simulink subsystem "forward_wheel"  (R2024b)
settings: Solver=VariableStepAuto  StartTime=0.0  StopTime=10.0  RelTol=1e-3
undefined symbols (not defined in the file): C_i, J, min_velocity, R
settings Model: Creator=Yevgeniy Gorbachev  LastModifiedBy=Yevgeniy Gorbachev

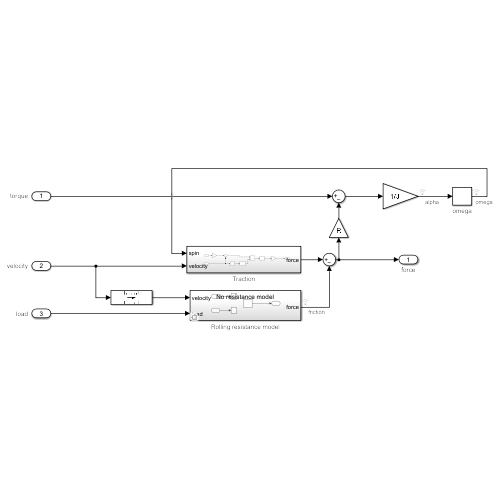
[thumbnail: Simulink's stored preview of the top-level diagram]
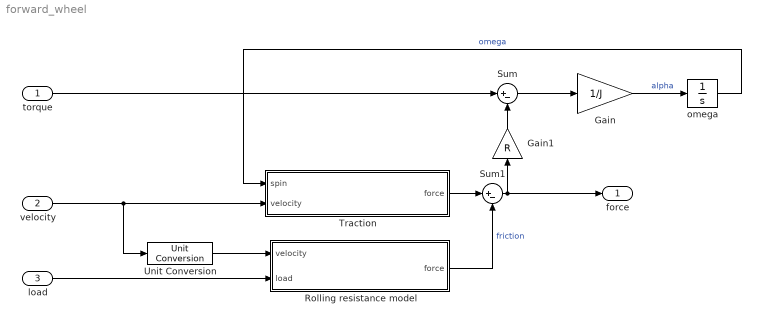
== system forward_wheel ==
  torque : Inport  Unit=N*m@torque  PortDimensions=1
  velocity : Inport  Port=2  Unit=m/s  PortDimensions=1
  load : Inport  Port=3  Unit=N  PortDimensions=1
  Gain : Gain  Gain=1/J
  Gain1 : Gain  Gain=R
  Rolling resistance model : Subsystem  Variant=on  VariantControl=Rolling resistance model
  Sum : Sum  Inputs=|+-
  Sum1 : Sum  Inputs=|+-
  Traction : Subsystem
  Unit Conversion : UnitConversion
  omega : Integrator  InitialCondition=10/R*0
  force : Outport  Unit=N  PortDimensions=1
  wires:
  Sum/1 -> Gain/1
  Gain/1 -> omega/1  "alpha"
  torque/1 -> Sum/1
  velocity/1 -> Unit Conversion/1, Traction/2(velocity)
  omega/1 -> Traction/1(spin)  "omega"
  Gain1/1 -> Sum/2
  Traction/1(force) -> Sum1/1
  Sum1/1 -> Gain1/1, force/1
  Unit Conversion/1 -> Rolling resistance model/1(velocity)
  load/1 -> Rolling resistance model/2(load)
  Rolling resistance model/1(force) -> Sum1/2  "friction"

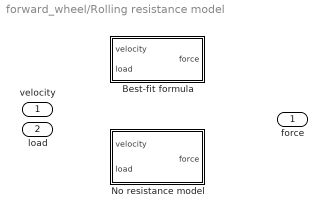
== system forward_wheel/Rolling resistance model ==
  velocity : Inport
  load : Inport  Port=2
  Best-fit formula : Subsystem  VariantControl=friction == true
  No resistance model : Subsystem  VariantControl=friction == false
  force : Outport

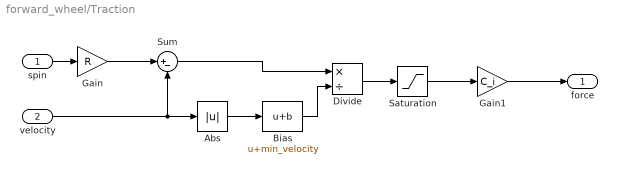
== system forward_wheel/Traction ==
  spin : Inport  Unit=rad/s
  velocity : Inport  Port=2  Unit=m/s
  Abs : Abs  SaturateOnIntegerOverflow=off
  Bias : Bias  Bias=min_velocity  SaturateOnIntegerOverflow=off
  Divide : Product  Inputs=*/
  Gain : Gain  Gain=R
  Gain1 : Gain  Gain=C_i
  Saturation : Saturate  UpperLimit=0.05  LowerLimit=-0.05
  Sum : Sum  Inputs=|+-
  force : Outport  Unit=N
  wires:
  Divide/1 -> Saturation/1
  Sum/1 -> Divide/1
  Bias/1 -> Divide/2
  Abs/1 -> Bias/1
  Gain/1 -> Sum/1
  Saturation/1 -> Gain1/1
  Gain1/1 -> force/1
  spin/1 -> Gain/1
  velocity/1 -> Sum/2, Abs/1

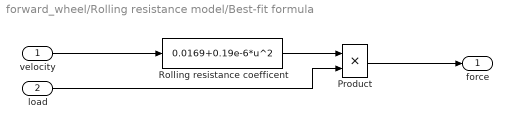
== system forward_wheel/Rolling resistance model/Best-fit formula ==
  velocity : Inport  Unit=km/h
  load : Inport  Port=2  Unit=N
  Product : Product
  Rolling resistance coefficent : Fcn  Expr=0.0169+0.19e-6*u^2
  force : Outport  Unit=N
  wires:
  velocity/1 -> Rolling resistance coefficent/1
  Product/1 -> force/1
  Rolling resistance coefficent/1 -> Product/1
  load/1 -> Product/2

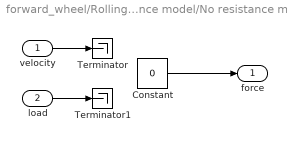
== system forward_wheel/Rolling resistance model/No resistance model ==
  velocity : Inport  Unit=km/h
  load : Inport  Port=2  Unit=N
  Constant : Constant  Value=0
  Terminator : Terminator
  Terminator1 : Terminator
  force : Outport  Unit=N
  wires:
  Constant/1 -> force/1
  load/1 -> Terminator1/1
  velocity/1 -> Terminator/1
